simulink model "Triple_rotor_Tilerotor_model"  (R2024b)
settings: Solver=ode45  StartTime=0.0  StopTime=100  FixedStep=1e-3  RelTol=1e-3
values from neighbouring files (symbols this model uses):
  para =     [Triple_Rotors_Tilrotor_Parameters.mat]
undefined symbols (not defined in the file or in its folder): initial_height, initial_pitch, initial_vx, magnitude, rot2
libraries: simulink x9, slpidlib x5, matrix_library x4, vrlib x1
(part 1 of 3)
settings Model: Creator=18336  LastModifiedBy=18336
settings OptimizationCC: ReuseModelBlockBuffer=off
settings RTWCC: GPUComputeCapability=3.5

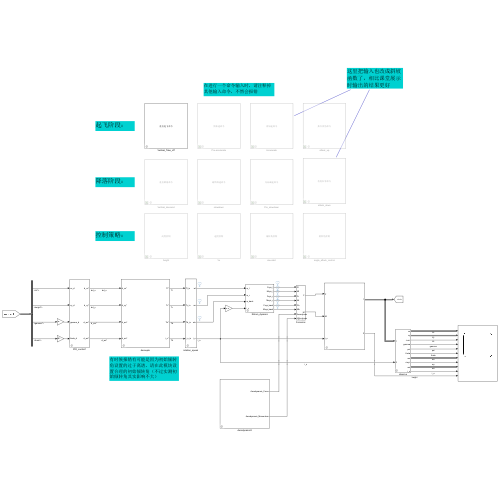
[thumbnail: Simulink's stored preview of the top-level diagram]
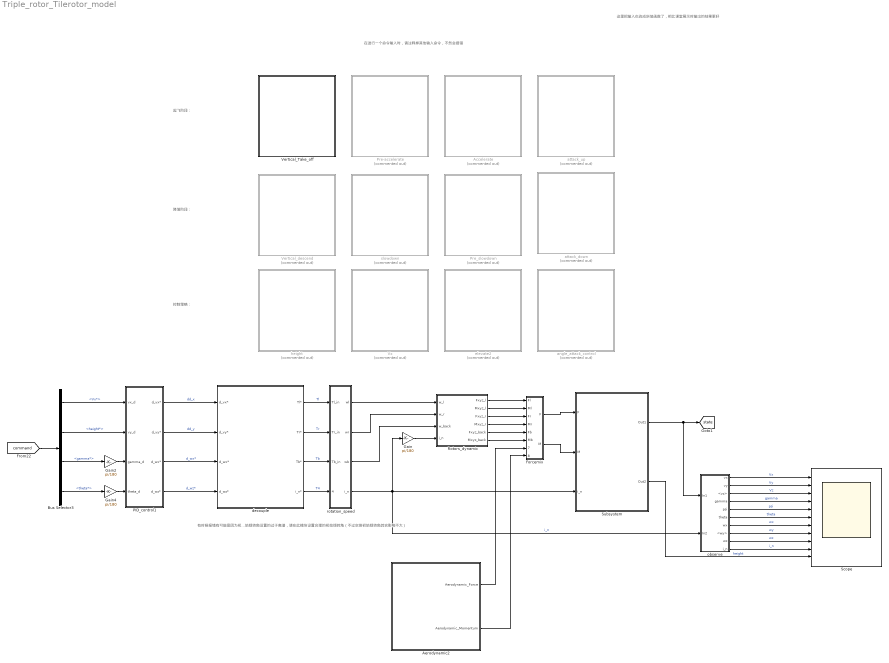
== system Triple_rotor_Tilerotor_model ==
  note: 这里把输入也改成斜坡函数了，相比课堂展示时输出的结果更好
  note: 在进行一个命令输入时，请注释掉其他输入命令，不然会报错
  note: 有时候报错有可能是因为初始倾转角设置的过于离谱，请在此模块设置合理的初始倾转角（不过实测初始倾转角其实影响不大）
  note: 起飞阶段：
  note: 降落阶段：
  note: 控制策略：
  Accelerate : Subsystem  Commented=on  mask{final_velocity=100, slope=10, Aerodynamic_switch=1}
      mask prompts: final_velocity "最终速度（m/s）"; slope "输入斜率"; Aerodynamic_switch "气动开关"
      mask DialogControl ParameterGroupVar Prompt: 参数
      mask Display: disp('再加速命令');
  Aerodynamic2 : Subsystem
  Bus Selector3 : BusSelector  OutputSignals=Vx*,height*,gamma*,theta*
  Forcemix : Subsystem
  Gain : Gain  Gain=pi/180
  Gain2 : Gain  Gain=pi/180
  Gain4 : Gain  Gain=pi/180
  PID_control1 : Subsystem  mask{P_d_vx=2, I_d_vx=1.3, D_d_vx=0, P_y=0.6, P_d_vy=1, I_d_vy=1.4, D_d_vy=0.1, P_wx=1, P_d_wx=1, I_d_wx=0, D_d_wx=0, P_wz=8, I_wz=2, D_wz=0, P_d_wz=6, I_d_wz=2, D_d_wz=8}
      mask prompts: P_d_vx "位置增益"; I_d_vx "积分增益"; D_d_vx "微分增益"; P_y "位置增益"; P_d_vy "速度位置增益"; I_d_vy "速度积分增益"; D_d_vy "速度微分增益"; P_wx "位置增益"; P_d_wx "二级位置增益"; I_d_wx "二级积分增益"; D_d_wx "二级微分增益"; P_wz "位置增益"; I_wz "积分增益"; D_wz "微分增益"; P_d_wz "二级位置增益"; I_d_wz "二级积分增益"; D_d_wz "二级微分增益"
      mask DialogControl ParameterGroupVar Prompt: 参数
      mask DialogControl x Prompt: x方向速度控制参数
      mask DialogControl y Prompt: y方向速度控制参数
      mask DialogControl wx Prompt: x方向角速度控制参数
      mask DialogControl wz Prompt: z方向角速度控制参数
  Pre-accelerate : Subsystem  Commented=on  mask{final_velocity=30, Aerodynamic_switch=0}
      mask prompts: final_velocity "最终速度（m/s）"; Aerodynamic_switch "气动开关"
      mask DialogControl ParameterGroupVar Prompt: 参数
      mask Display: disp('预加速命令');
  Pre_slowdown : Subsystem  Commented=on  mask{initial_velocity=100, Aerodynamic_switch=1}
      mask prompts: initial_velocity "初始速度（m/s）"; Aerodynamic_switch "气动开关"
      mask DialogControl ParameterGroupVar Prompt: 参数
      mask Display: disp('反向减速命令');
  Rotors_dynamic : Subsystem
  Scope : Scope  NumInputPorts=11
  Subsystem : Subsystem
  Vertical_Take_off : Subsystem  mask{slope_y=20, max_y=1000, Aerodynamic_switch=0}
      mask prompts: slope_y "上升速度（m/s）"; max_y "最终高度（m）"; Aerodynamic_switch "气动开关"
      mask DialogControl ParameterGroupVar Prompt: 参数
      mask Display: disp('垂直起飞命令');
  Vertical_descend : Subsystem  Commented=on  mask{slope_y=20, initial_y=1000, Aerodynamic_switch=0}
      mask prompts: slope_y "下降速度（m/s）"; initial_y "初始高度（m）"; Aerodynamic_switch "气动开关"
      mask DialogControl ParameterGroupVar Prompt: 参数
      mask Display: disp('垂直降落命令');
  Vx : Subsystem  Commented=on  mask{final_velocity=110, slope=10, Aerodynamic_switch=1}
      mask prompts: final_velocity "最终速度（m/s）"; slope "斜率"; Aerodynamic_switch "气动开关"
      mask DialogControl ParameterGroupVar Prompt: 参数
      mask Display: disp('速度控制');
  angle_attack_control : Subsystem  Commented=on  mask{final_theta=-2, slope=-2, Aerodynamic_switch=1}
      mask prompts: final_theta "最终俯仰角度"; slope "斜率"; Aerodynamic_switch "气动开关"
      mask DialogControl ParameterGroupVar Prompt: 参数
      mask Display: disp('俯仰角控制');
  attack_down : Subsystem  Commented=on  mask{initial_theta=4, slope=-1, Aerodynamic_switch=1}
      mask prompts: initial_theta "初始俯仰角"; slope "输入斜率"; Aerodynamic_switch "气动开关"
      mask DialogControl ParameterGroupVar Prompt: 参数
      mask Display: disp('攻角归零命令');
  attack_up : Subsystem  Commented=on  mask{final_theta=4, Aerodynamic_switch=1}
      mask prompts: final_theta "最终俯仰角"; Aerodynamic_switch "气动开关"
      mask DialogControl ParameterGroupVar Prompt: 参数
      mask Display: disp('抬升攻角命令');
  decouple : Subsystem  mask{initial_i_n=30}
      mask prompts: initial_i_n "初始短仓角"
      mask DialogControl ParameterGroupVar Prompt: 参数
  elevate2 : Subsystem  Commented=on  mask{max_gamma=4, slope=8, Aerodynamic_switch=0}
      mask prompts: max_gamma "最大滚转角°"; slope "斜率"; Aerodynamic_switch "气动开关"
      mask DialogControl ParameterGroupVar Prompt: 参数
      mask Display: disp('滚转角控制');
  height : Subsystem  Commented=on  mask{final_y=1100, slope=10, Aerodynamic_switch=1}
      mask prompts: final_y "最终高度"; slope "变化速度"; Aerodynamic_switch "气动开关"
      mask DialogControl ParameterGroupVar Prompt: 参数
      mask Display: disp('高度控制');
  observe : Subsystem
  rotation_speed : Subsystem  mask{maxrot=para.maxrot, minrot=1, maxi_n=170, mini_n=10}
      mask prompts: maxrot "旋翼最大转速"; minrot "旋翼最小转速"
      mask DialogControl ParameterGroupVar Prompt: 参数
  slowdown : Subsystem  Commented=on  mask{initial_velocity=30, Aerodynamic_switch=0}
      mask prompts: initial_velocity "初始速度（m/s）"; Aerodynamic_switch "气动开关"
      mask DialogControl ParameterGroupVar Prompt: 参数
      mask Display: disp('最终降速命令');
  tag scope: state=global
  wires:
  Subsystem/1(Out1) -> observe/1(In1), [state]
  rotation_speed/4(i_n) -> observe/2(In2), Subsystem/3(i_n), Gain/1  "i_n"
  Gain/1 -> Rotors_dynamic/4(i_n)
  Bus Selector3/2 -> PID_control1/2(vy_d)  "<height*>"
  PID_control1/1(d_vx*) -> decouple/1(d_vx*)  "dd_x"
  PID_control1/2(d_vy*) -> decouple/2(d_vy*)  "dd_y"
  PID_control1/3(d_wx*) -> decouple/3(d_wx*)  "d_wx*"
  PID_control1/4(d_wz*) -> decouple/4(d_wz*)  "d_wz*"
  Rotors_dynamic/4(Mxyz_r) -> Forcemix/4(Mr)
  Rotors_dynamic/1(Fxyz_l) -> Forcemix/1(Fl)
  Rotors_dynamic/2(Mxyz_l) -> Forcemix/2(Ml)
  Rotors_dynamic/6(Mxyz_back) -> Forcemix/6(Mb)
  rotation_speed/1(wl) -> Rotors_dynamic/1(w_l)
  rotation_speed/2(wr) -> Rotors_dynamic/2(w_r)
  rotation_speed/3(wb) -> Rotors_dynamic/3(w_back)
  Forcemix/1(F) -> Subsystem/1(F)
  Bus Selector3/3 -> Gain2/1  "<gamma*>"
  Rotors_dynamic/3(Fxyz_r) -> Forcemix/3(Fr)
  Rotors_dynamic/5(Fxyz_back) -> Forcemix/5(Fb)
  Aerodynamic2/1(Aerodynamic_Force) -> Forcemix/7(Aerodynamic_Force)
  Aerodynamic2/2(Aerodynamic_Momentum) -> Forcemix/8(Aerodynamic_Momentum)
  Gain4/1 -> PID_control1/4(theta_d)
  Forcemix/2(M) -> Subsystem/2(M)
  decouple/3(Tb*) -> rotation_speed/3(Tb_in)  "Tb"
  decouple/2(Tr*) -> rotation_speed/2(Tr_in)  "Tr"
  decouple/1(Tl*) -> rotation_speed/1(Tl_in)  "Tl"
  decouple/4(i_n*) -> rotation_speed/4(i_n_in)  "T4"
  Gain2/1 -> PID_control1/3(gamma_d)
  Subsystem/2(Out2) -> Scope/11  "height"
  [command] -> Bus Selector3/1
  Bus Selector3/1 -> PID_control1/1(vx_d)  "<Vx*>"
  Bus Selector3/4 -> Gain4/1  "<theta*>"
  observe/1(vx) -> Scope/1  "Vx"
  observe/2(vy) -> Scope/2  "Vy"
  observe/3(<vz>) -> Scope/3  "Vz"
  observe/4(gamma) -> Scope/4  "gamma"
  observe/5(psi) -> Scope/5  "psi"
  observe/6(theta) -> Scope/6  "theta"
  observe/7(wx) -> Scope/7  "wx"
  observe/8(<wy>) -> Scope/8  "wy"
  observe/9(wz) -> Scope/9  "wz"
  observe/10(i_n) -> Scope/10  "i_n"

== system Triple_rotor_Tilerotor_model/Accelerate ==
  note: 阶跃输入请用这个
  Bus Creator : BusCreator  Inputs=4
  Constant : Constant  Value=Aerodynamic_switch
  Constant1 : Constant  Value=0
  Constant2 : Constant  Value=1000
  Constant3 : Constant  Value=0
  Constant4 : Constant  Value=30
  Ramp : simulink/Sources/Ramp  slope=slope  start=0  InitialOutput=30
  Saturation2 : Saturate  UpperLimit=final_velocity  LowerLimit=0
  Step : Step  Commented=on  Time=0  Before=30  After=final_velocity  SampleTime=0
  gamma* : Constant  Value=0
  height : Constant  Value=1000
  theta* : Constant  Value=0
  tag scope: Aerodynamic_switch=global, command=global, initial_Vx=global, initial_gamma=global, initial_height=global, initial_theta=global
  wires:
  theta*/1 -> Bus Creator/4  "theta*"
  height/1 -> Bus Creator/2  "height*"
  gamma*/1 -> Bus Creator/3  "gamma*"
  Saturation2/1 -> Bus Creator/1  "Vx*"
  Bus Creator/1 -> [command]
  Constant/1 -> [Aerodynamic_switch]
  Constant1/1 -> [initial_theta]
  Constant3/1 -> [initial_gamma]
  Constant2/1 -> [initial_height]
  Constant4/1 -> [initial_Vx]
  Ramp/1 -> Saturation2/1

== system Triple_rotor_Tilerotor_model/Aerodynamic2 ==
  Aerodynamic Modal of Horizontal Stabilizer : Subsystem
  Aerodynamic Modal of the Left Verticall Stabilizer : Subsystem
  Aerodynamic Modal of the Right Verticall Stabilizer : Subsystem
  Aerodynamic Model of the Fuselage : Subsystem
  Aerodynamic Model of the Wing : Subsystem
  Demux{,1..3} (4 alike) : Demux  Outputs=3
  Product : Product
  Product1 : Product
  Resultant Force : Sum  Inputs=+++++
  Resultant Moment : Sum  Inputs=+++++
  Scope1 : Scope  NumInputPorts=3
  Scope2 : Scope  NumInputPorts=3
  Aerodynamic_Force : Outport
  Aerodynamic_Momentum : Outport  Port=2
  tag scope: Fx_forward=global, Fy_forward=global, Mx_forward=global, Mz_forward=global
  wires:
  [state] -> Aerodynamic Model of the Wing/1(In1)
  [state] -> Aerodynamic Model of the Fuselage/1(In1)
  Aerodynamic Modal of Horizontal Stabilizer/2(Vector of Momentum in Center of Gravity) -> Resultant Moment/3
  Aerodynamic Model of the Wing/2(Momentum of Wing Output) -> Resultant Moment/1
  Aerodynamic Modal of the Right Verticall Stabilizer/1(Out1) -> Resultant Force/5
  Aerodynamic Model of the Fuselage/1(Force of Fuselage) -> Resultant Force/3
  [state] -> Aerodynamic Modal of the Left Verticall Stabilizer/1(In1)
  Aerodynamic Modal of Horizontal Stabilizer/1(Vector of Force in Center of Gravity) -> Resultant Force/1
  [state] -> Aerodynamic Modal of the Right Verticall Stabilizer/1(In1)
  Aerodynamic Modal of the Right Verticall Stabilizer/2(Out2) -> Resultant Moment/5
  Aerodynamic Modal of the Left Verticall Stabilizer/2(Out2) -> Resultant Moment/4
  [state] -> Aerodynamic Modal of Horizontal Stabilizer/1(In1)
  Aerodynamic Modal of the Left Verticall Stabilizer/1(Out1) -> Resultant Force/4
  Aerodynamic Model of the Fuselage/2(Momentum of Fuselage) -> Resultant Moment/2
  Aerodynamic Model of the Wing/1(Force of Wing Output) -> Resultant Force/2
  Product/1 -> Demux2/1, Demux/1, Aerodynamic_Force/1
  Demux/1 -> [Fx_forward]
  Demux/2 -> [Fy_forward]
  Demux1/1 -> [Mx_forward]
  Demux1/3 -> [Mz_forward]
  Resultant Force/1 -> Product/1
  Resultant Moment/1 -> Product1/1
  Demux2/1 -> Scope1/1
  Demux2/2 -> Scope1/2
  Demux2/3 -> Scope1/3
  Demux3/1 -> Scope2/1
  Demux3/2 -> Scope2/2
  Product1/1 -> Demux3/1, Demux1/1, Aerodynamic_Momentum/1
  Demux3/3 -> Scope2/3
  [Aerodynamic_switch] -> Product1/2, Product/2

== system Triple_rotor_Tilerotor_model/Forcemix ==
  Fl : Inport
  Ml : Inport  Port=2
  Fr : Inport  Port=3
  Mr : Inport  Port=4
  Fb : Inport  Port=5
  Mb : Inport  Port=6
  Aerodynamic_Force : Inport  Port=7
  Aerodynamic_Momentum : Inport  Port=8
  Demux : Demux  Outputs=3
  Demux1 : Demux  Outputs=3
  Goto : Goto  Commented=on  GotoTag=F  TagVisibility=global
  Goto1 : Goto  Commented=on  GotoTag=M
  Scope1 : Scope  NumInputPorts=6
  rotor_forcemix : Subsystem
  F : Outport
  M : Outport  Port=2
  wires:
  Demux1/3 -> Scope1/6  "Mz"
  Demux1/1 -> Scope1/4  "Mx"
  Demux1/2 -> Scope1/5  "My"
  Demux/1 -> Scope1/1  "Fx"
  Demux/2 -> Scope1/2  "Fy"
  Demux/3 -> Scope1/3  "Fz"
  Fr/1 -> rotor_forcemix/3(Fr)
  Mr/1 -> rotor_forcemix/4(Mr)
  Fl/1 -> rotor_forcemix/1(Fl)
  Ml/1 -> rotor_forcemix/2(Ml)
  Fb/1 -> rotor_forcemix/5(Fb)
  Mb/1 -> rotor_forcemix/6(Mb)
  rotor_forcemix/1(Out1) -> F/1, Demux/1
  rotor_forcemix/2(Out2) -> Demux1/1, M/1
  Aerodynamic_Force/1 -> rotor_forcemix/7(AF)
  Aerodynamic_Momentum/1 -> rotor_forcemix/8(AM)

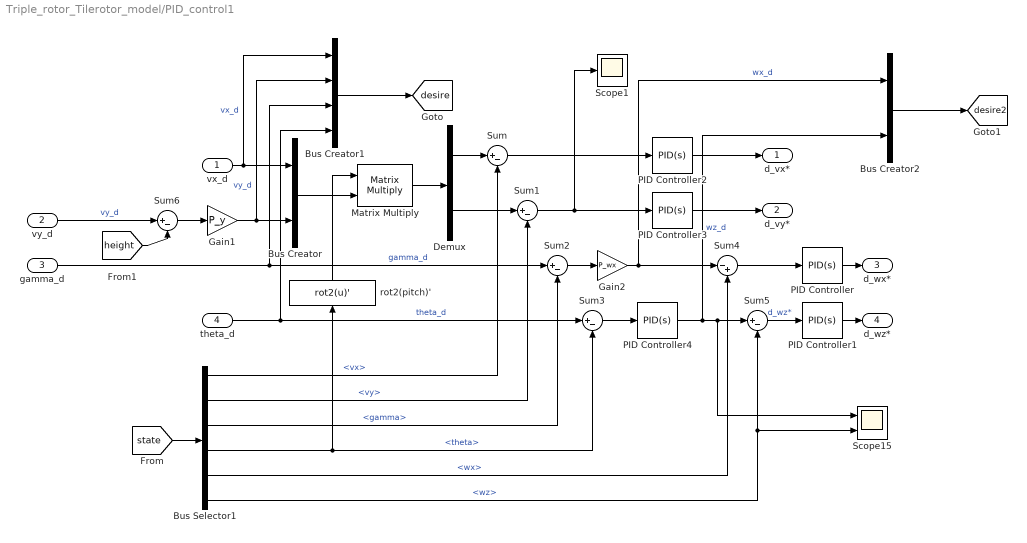
== system Triple_rotor_Tilerotor_model/PID_control1 ==
  vx_d : Inport
  vy_d : Inport  Port=2
  gamma_d : Inport  Port=3
  theta_d : Inport  Port=4
  Bus Creator : BusCreator  Inputs=2
  Bus Creator1 : BusCreator  Inputs=4
  Bus Creator2 : BusCreator  Inputs=2
  Bus Selector1 : BusSelector  OutputSignals=vx,vy,gamma,theta,wx,wz
  Demux : Demux  Outputs=2
  Gain1 : Gain  Gain=P_y
  Gain2 : Gain  Gain=P_wx
  Matrix Multiply : Product  Multiplication=Matrix(*)
  PID Controller : slpidlib/PID Controller  Controller=PID  Form=Parallel  TimeDomain=Continuous-time  UseExternalTs=off  SampleTime=-1  IntegratorMethod=Forward Euler  FilterMethod=Forward Euler  ControllerParametersSource=internal  P=P_d_wx  I=I_d_wx  UseKiTs=off  D=D_d_wx  UseExternalDerivativeSource=off  N=100  UseFilter=on  TunerSelectOption=Transfer Function Based (PID Tuner App)  InitialConditionSource=internal  InitialConditionForIntegrator=0  InitialConditionForFilter=0  DifferentiatorICPrevScaledInput=0  ExternalReset=none  TrackingMode=off  Kt=1  LimitOutput=off  SatLimitsSource=internal  UpperSaturationLimit=inf  LowerSaturationLimit=-inf  LinearizeAsGain=on  AntiWindupMode=none  Kb=1  LimitIntegrator=off  UpperIntegratorSaturationLimit=inf  LowerIntegratorSaturationLimit=-inf  POutMin=[]  POutMax=[]  IOutMin=[]  IOutMax=[]  DOutMin=[]  DOutMax=[]  NOutMin=[]  NOutMax=[]  SumOutMin=[]  SumOutMax=[]  SaturationOutMin=[]  SaturationOutMax=[]  PParamMin=[]  PParamMax=[]  IParamMin=[]  IParamMax=[]  DParamMin=[]  DParamMax=[]  NParamMin=[]  NParamMax=[]  KbParamMin=[]  KbParamMax=[]  KtParamMin=[]  KtParamMax=[]  KbOutMin=[]  KbOutMax=[]  KtOutMin=[]  KtOutMax=[]  IntegratorOutMin=[]  IntegratorOutMax=[]  FilterOutMin=[]  FilterOutMax=[]  SumI1OutMin=[]  SumI1OutMax=[]  SumI2OutMin=[]  SumI2OutMax=[]  SumI3OutMin=[]  SumI3OutMax=[]  SumI4OutMin=[]  SumI4OutMax=[]  SumDOutMin=[]  SumDOutMax=[]  DifferentiatorOutMin=[]  DifferentiatorOutMax=[]  FilterDiffOutCoefMin=[]  FilterDiffOutCoefMax=[]  ReciprocalOutMin=[]  ReciprocalOutMax=[]  SumDenOutMin=[]  SumDenOutMax=[]  SumNumOutMin=[]  SumNumOutMax=[]  DivideOutMin=[]  DivideOutMax=[]  UdiffTsProdOutMin=[]  UdiffTsProdOutMax=[]  NTsProdOutMin=[]  NTsProdOutMax=[]  UintegralTsProdOutMin=[]  UintegralTsProdOutMax=[]  UngainTsProdOutMin=[]  UngainTsProdOutMax=[]  ClampingZeroOutDataTypeStr=Inherit: Inherit via back propagation  ClampingZeroOutMin=[]  ClampingZeroOutMax=[]  FilterDenConstantOutDataTypeStr=Inherit: Inherit via back propagation  FilterDenConstantOutMin=[]  FilterDenConstantOutMax=[]  PCopyOutDataTypeStr=Inherit: Inherit via back propagation  PCopyOutMin=[]  PCopyOutMax=[]  NCopyOutDataTypeStr=Inherit: Inherit via back propagation  NCopyOutMin=[]  NCopyOutMax=[]  IntegratorContinuousStateAttributes=''  IntegratorStateMustResolveToSignalObject=off  IntegratorRTWStateStorageClass=Auto  FilterContinuousStateAttributes=''  FilterStateMustResolveToSignalObject=off  FilterRTWStateStorageClass=Auto  ParallelPVariant=InternalParameters  IdealPVariant=Disabled  IVariant=InternalParameters  DVariant=InternalParameters  IntegratorVariant=Continuous  SatVariant=Disabled  AWVariant=Passthrough  PCopyVariant=Disabled  TRVariant=Disabled  FdbkBlocksVariant=Forward  IdealPFdbkVariant=Disabled  SatFdbkVariant=Disabled  DerivativeFilterVariant=ContFilter  NVariant=InternalParameters  NCopyVariant=Disabled  FilterICVariant=InternalICsFilter  IntegratorICVariant=InternalICs  ExternalResetVariant=Disabled  TRSumVariant=Passthrough  SumFdbkVariant=Disabled  SumVariant=Sum_PID  TsampFilterVariant=InternalTs  TsampNgainVariant=Passthrough  TsampIntegralVariant=Disabled_SignalSpec  ExternalSaturationOutDataTypeStr=Inherit: Same as second input  DerivativeSourceVariant=ErrorSignal  PreIntVariant=InternalPreInt
  PID Controller1 : slpidlib/PID Controller  Controller=PID  Form=Parallel  TimeDomain=Continuous-time  UseExternalTs=off  SampleTime=-1  IntegratorMethod=Forward Euler  FilterMethod=Forward Euler  ControllerParametersSource=internal  P=P_d_wz  I=I_d_wz  UseKiTs=off  D=D_d_wz  UseExternalDerivativeSource=off  N=100  UseFilter=on  TunerSelectOption=Transfer Function Based (PID Tuner App)  InitialConditionSource=internal  InitialConditionForIntegrator=0  InitialConditionForFilter=0  DifferentiatorICPrevScaledInput=0  ExternalReset=none  TrackingMode=off  Kt=1  LimitOutput=off  SatLimitsSource=internal  UpperSaturationLimit=inf  LowerSaturationLimit=-inf  LinearizeAsGain=on  AntiWindupMode=none  Kb=1  LimitIntegrator=off  UpperIntegratorSaturationLimit=inf  LowerIntegratorSaturationLimit=-inf  POutMin=[]  POutMax=[]  IOutMin=[]  IOutMax=[]  DOutMin=[]  DOutMax=[]  NOutMin=[]  NOutMax=[]  SumOutMin=[]  SumOutMax=[]  SaturationOutMin=[]  SaturationOutMax=[]  PParamMin=[]  PParamMax=[]  IParamMin=[]  IParamMax=[]  DParamMin=[]  DParamMax=[]  NParamMin=[]  NParamMax=[]  KbParamMin=[]  KbParamMax=[]  KtParamMin=[]  KtParamMax=[]  KbOutMin=[]  KbOutMax=[]  KtOutMin=[]  KtOutMax=[]  IntegratorOutMin=[]  IntegratorOutMax=[]  FilterOutMin=[]  FilterOutMax=[]  SumI1OutMin=[]  SumI1OutMax=[]  SumI2OutMin=[]  SumI2OutMax=[]  SumI3OutMin=[]  SumI3OutMax=[]  SumI4OutMin=[]  SumI4OutMax=[]  SumDOutMin=[]  SumDOutMax=[]  DifferentiatorOutMin=[]  DifferentiatorOutMax=[]  FilterDiffOutCoefMin=[]  FilterDiffOutCoefMax=[]  ReciprocalOutMin=[]  ReciprocalOutMax=[]  SumDenOutMin=[]  SumDenOutMax=[]  SumNumOutMin=[]  SumNumOutMax=[]  DivideOutMin=[]  DivideOutMax=[]  UdiffTsProdOutMin=[]  UdiffTsProdOutMax=[]  NTsProdOutMin=[]  NTsProdOutMax=[]  UintegralTsProdOutMin=[]  UintegralTsProdOutMax=[]  UngainTsProdOutMin=[]  UngainTsProdOutMax=[]  ClampingZeroOutDataTypeStr=Inherit: Inherit via back propagation  ClampingZeroOutMin=[]  ClampingZeroOutMax=[]  FilterDenConstantOutDataTypeStr=Inherit: Inherit via back propagation  FilterDenConstantOutMin=[]  FilterDenConstantOutMax=[]  PCopyOutDataTypeStr=Inherit: Inherit via back propagation  PCopyOutMin=[]  PCopyOutMax=[]  NCopyOutDataTypeStr=Inherit: Inherit via back propagation  NCopyOutMin=[]  NCopyOutMax=[]  IntegratorContinuousStateAttributes=''  IntegratorStateMustResolveToSignalObject=off  IntegratorRTWStateStorageClass=Auto  FilterContinuousStateAttributes=''  FilterStateMustResolveToSignalObject=off  FilterRTWStateStorageClass=Auto  ParallelPVariant=InternalParameters  IdealPVariant=Disabled  IVariant=InternalParameters  DVariant=InternalParameters  IntegratorVariant=Continuous  SatVariant=Disabled  AWVariant=Passthrough  PCopyVariant=Disabled  TRVariant=Disabled  FdbkBlocksVariant=Forward  IdealPFdbkVariant=Disabled  SatFdbkVariant=Disabled  DerivativeFilterVariant=ContFilter  NVariant=InternalParameters  NCopyVariant=Disabled  FilterICVariant=InternalICsFilter  IntegratorICVariant=InternalICs  ExternalResetVariant=Disabled  TRSumVariant=Passthrough  SumFdbkVariant=Disabled  SumVariant=Sum_PID  TsampFilterVariant=InternalTs  TsampNgainVariant=Passthrough  TsampIntegralVariant=Disabled_SignalSpec  ExternalSaturationOutDataTypeStr=Inherit: Same as second input  DerivativeSourceVariant=ErrorSignal  PreIntVariant=InternalPreInt
  PID Controller2 : slpidlib/PID Controller  Controller=PID  Form=Parallel  TimeDomain=Continuous-time  UseExternalTs=off  SampleTime=-1  IntegratorMethod=Forward Euler  FilterMethod=Forward Euler  ControllerParametersSource=internal  P=P_d_vx  I=I_d_vx  UseKiTs=off  D=D_d_vx  UseExternalDerivativeSource=off  N=100  UseFilter=on  TunerSelectOption=Transfer Function Based (PID Tuner App)  InitialConditionSource=internal  InitialConditionForIntegrator=0  InitialConditionForFilter=0  DifferentiatorICPrevScaledInput=0  ExternalReset=none  TrackingMode=off  Kt=1  LimitOutput=off  SatLimitsSource=internal  UpperSaturationLimit=inf  LowerSaturationLimit=-inf  LinearizeAsGain=on  AntiWindupMode=none  Kb=1  LimitIntegrator=off  UpperIntegratorSaturationLimit=inf  LowerIntegratorSaturationLimit=-inf  POutMin=[]  POutMax=[]  IOutMin=[]  IOutMax=[]  DOutMin=[]  DOutMax=[]  NOutMin=[]  NOutMax=[]  SumOutMin=[]  SumOutMax=[]  SaturationOutMin=[]  SaturationOutMax=[]  PParamMin=[]  PParamMax=[]  IParamMin=[]  IParamMax=[]  DParamMin=[]  DParamMax=[]  NParamMin=[]  NParamMax=[]  KbParamMin=[]  KbParamMax=[]  KtParamMin=[]  KtParamMax=[]  KbOutMin=[]  KbOutMax=[]  KtOutMin=[]  KtOutMax=[]  IntegratorOutMin=[]  IntegratorOutMax=[]  FilterOutMin=[]  FilterOutMax=[]  SumI1OutMin=[]  SumI1OutMax=[]  SumI2OutMin=[]  SumI2OutMax=[]  SumI3OutMin=[]  SumI3OutMax=[]  SumI4OutMin=[]  SumI4OutMax=[]  SumDOutMin=[]  SumDOutMax=[]  DifferentiatorOutMin=[]  DifferentiatorOutMax=[]  FilterDiffOutCoefMin=[]  FilterDiffOutCoefMax=[]  ReciprocalOutMin=[]  ReciprocalOutMax=[]  SumDenOutMin=[]  SumDenOutMax=[]  SumNumOutMin=[]  SumNumOutMax=[]  DivideOutMin=[]  DivideOutMax=[]  UdiffTsProdOutMin=[]  UdiffTsProdOutMax=[]  NTsProdOutMin=[]  NTsProdOutMax=[]  UintegralTsProdOutMin=[]  UintegralTsProdOutMax=[]  UngainTsProdOutMin=[]  UngainTsProdOutMax=[]  ClampingZeroOutDataTypeStr=Inherit: Inherit via back propagation  ClampingZeroOutMin=[]  ClampingZeroOutMax=[]  FilterDenConstantOutDataTypeStr=Inherit: Inherit via back propagation  FilterDenConstantOutMin=[]  FilterDenConstantOutMax=[]  PCopyOutDataTypeStr=Inherit: Inherit via back propagation  PCopyOutMin=[]  PCopyOutMax=[]  NCopyOutDataTypeStr=Inherit: Inherit via back propagation  NCopyOutMin=[]  NCopyOutMax=[]  IntegratorContinuousStateAttributes=''  IntegratorStateMustResolveToSignalObject=off  IntegratorRTWStateStorageClass=Auto  FilterContinuousStateAttributes=''  FilterStateMustResolveToSignalObject=off  FilterRTWStateStorageClass=Auto  ParallelPVariant=InternalParameters  IdealPVariant=Disabled  IVariant=InternalParameters  DVariant=InternalParameters  IntegratorVariant=Continuous  SatVariant=Disabled  AWVariant=Passthrough  PCopyVariant=Disabled  TRVariant=Disabled  FdbkBlocksVariant=Forward  IdealPFdbkVariant=Disabled  SatFdbkVariant=Disabled  DerivativeFilterVariant=ContFilter  NVariant=InternalParameters  NCopyVariant=Disabled  FilterICVariant=InternalICsFilter  IntegratorICVariant=InternalICs  ExternalResetVariant=Disabled  TRSumVariant=Passthrough  SumFdbkVariant=Disabled  SumVariant=Sum_PID  TsampFilterVariant=InternalTs  TsampNgainVariant=Passthrough  TsampIntegralVariant=Disabled_SignalSpec  ExternalSaturationOutDataTypeStr=Inherit: Same as second input  DerivativeSourceVariant=ErrorSignal  PreIntVariant=InternalPreInt
  PID Controller3 : slpidlib/PID Controller  Controller=PID  Form=Parallel  TimeDomain=Continuous-time  UseExternalTs=off  SampleTime=-1  IntegratorMethod=Forward Euler  FilterMethod=Forward Euler  ControllerParametersSource=internal  P=P_d_vy  I=I_d_vy  UseKiTs=off  D=D_d_vy  UseExternalDerivativeSource=off  N=100  UseFilter=on  TunerSelectOption=Transfer Function Based (PID Tuner App)  InitialConditionSource=internal  InitialConditionForIntegrator=0  InitialConditionForFilter=0  DifferentiatorICPrevScaledInput=0  ExternalReset=none  TrackingMode=off  Kt=1  LimitOutput=off  SatLimitsSource=internal  UpperSaturationLimit=inf  LowerSaturationLimit=-inf  LinearizeAsGain=on  AntiWindupMode=none  Kb=1  LimitIntegrator=off  UpperIntegratorSaturationLimit=inf  LowerIntegratorSaturationLimit=-inf  POutMin=[]  POutMax=[]  IOutMin=[]  IOutMax=[]  DOutMin=[]  DOutMax=[]  NOutMin=[]  NOutMax=[]  SumOutMin=[]  SumOutMax=[]  SaturationOutMin=[]  SaturationOutMax=[]  PParamMin=[]  PParamMax=[]  IParamMin=[]  IParamMax=[]  DParamMin=[]  DParamMax=[]  NParamMin=[]  NParamMax=[]  KbParamMin=[]  KbParamMax=[]  KtParamMin=[]  KtParamMax=[]  KbOutMin=[]  KbOutMax=[]  KtOutMin=[]  KtOutMax=[]  IntegratorOutMin=[]  IntegratorOutMax=[]  FilterOutMin=[]  FilterOutMax=[]  SumI1OutMin=[]  SumI1OutMax=[]  SumI2OutMin=[]  SumI2OutMax=[]  SumI3OutMin=[]  SumI3OutMax=[]  SumI4OutMin=[]  SumI4OutMax=[]  SumDOutMin=[]  SumDOutMax=[]  DifferentiatorOutMin=[]  DifferentiatorOutMax=[]  FilterDiffOutCoefMin=[]  FilterDiffOutCoefMax=[]  ReciprocalOutMin=[]  ReciprocalOutMax=[]  SumDenOutMin=[]  SumDenOutMax=[]  SumNumOutMin=[]  SumNumOutMax=[]  DivideOutMin=[]  DivideOutMax=[]  UdiffTsProdOutMin=[]  UdiffTsProdOutMax=[]  NTsProdOutMin=[]  NTsProdOutMax=[]  UintegralTsProdOutMin=[]  UintegralTsProdOutMax=[]  UngainTsProdOutMin=[]  UngainTsProdOutMax=[]  ClampingZeroOutDataTypeStr=Inherit: Inherit via back propagation  ClampingZeroOutMin=[]  ClampingZeroOutMax=[]  FilterDenConstantOutDataTypeStr=Inherit: Inherit via back propagation  FilterDenConstantOutMin=[]  FilterDenConstantOutMax=[]  PCopyOutDataTypeStr=Inherit: Inherit via back propagation  PCopyOutMin=[]  PCopyOutMax=[]  NCopyOutDataTypeStr=Inherit: Inherit via back propagation  NCopyOutMin=[]  NCopyOutMax=[]  IntegratorContinuousStateAttributes=''  IntegratorStateMustResolveToSignalObject=off  IntegratorRTWStateStorageClass=Auto  FilterContinuousStateAttributes=''  FilterStateMustResolveToSignalObject=off  FilterRTWStateStorageClass=Auto  ParallelPVariant=InternalParameters  IdealPVariant=Disabled  IVariant=InternalParameters  DVariant=InternalParameters  IntegratorVariant=Continuous  SatVariant=Disabled  AWVariant=Passthrough  PCopyVariant=Disabled  TRVariant=Disabled  FdbkBlocksVariant=Forward  IdealPFdbkVariant=Disabled  SatFdbkVariant=Disabled  DerivativeFilterVariant=ContFilter  NVariant=InternalParameters  NCopyVariant=Disabled  FilterICVariant=InternalICsFilter  IntegratorICVariant=InternalICs  ExternalResetVariant=Disabled  TRSumVariant=Passthrough  SumFdbkVariant=Disabled  SumVariant=Sum_PID  TsampFilterVariant=InternalTs  TsampNgainVariant=Passthrough  TsampIntegralVariant=Disabled_SignalSpec  ExternalSaturationOutDataTypeStr=Inherit: Same as second input  DerivativeSourceVariant=ErrorSignal  PreIntVariant=InternalPreInt
  PID Controller4 : slpidlib/PID Controller  Controller=PID  Form=Parallel  TimeDomain=Continuous-time  UseExternalTs=off  SampleTime=-1  IntegratorMethod=Forward Euler  FilterMethod=Forward Euler  ControllerParametersSource=internal  P=P_wz  I=I_wz  UseKiTs=off  D=D_wz  UseExternalDerivativeSource=off  N=100  UseFilter=on  TunerSelectOption=Transfer Function Based (PID Tuner App)  InitialConditionSource=internal  InitialConditionForIntegrator=0  InitialConditionForFilter=0  DifferentiatorICPrevScaledInput=0  ExternalReset=none  TrackingMode=off  Kt=1  LimitOutput=off  SatLimitsSource=internal  UpperSaturationLimit=inf  LowerSaturationLimit=-inf  LinearizeAsGain=on  AntiWindupMode=none  Kb=1  LimitIntegrator=off  UpperIntegratorSaturationLimit=inf  LowerIntegratorSaturationLimit=-inf  POutMin=[]  POutMax=[]  IOutMin=[]  IOutMax=[]  DOutMin=[]  DOutMax=[]  NOutMin=[]  NOutMax=[]  SumOutMin=[]  SumOutMax=[]  SaturationOutMin=[]  SaturationOutMax=[]  PParamMin=[]  PParamMax=[]  IParamMin=[]  IParamMax=[]  DParamMin=[]  DParamMax=[]  NParamMin=[]  NParamMax=[]  KbParamMin=[]  KbParamMax=[]  KtParamMin=[]  KtParamMax=[]  KbOutMin=[]  KbOutMax=[]  KtOutMin=[]  KtOutMax=[]  IntegratorOutMin=[]  IntegratorOutMax=[]  FilterOutMin=[]  FilterOutMax=[]  SumI1OutMin=[]  SumI1OutMax=[]  SumI2OutMin=[]  SumI2OutMax=[]  SumI3OutMin=[]  SumI3OutMax=[]  SumI4OutMin=[]  SumI4OutMax=[]  SumDOutMin=[]  SumDOutMax=[]  DifferentiatorOutMin=[]  DifferentiatorOutMax=[]  FilterDiffOutCoefMin=[]  FilterDiffOutCoefMax=[]  ReciprocalOutMin=[]  ReciprocalOutMax=[]  SumDenOutMin=[]  SumDenOutMax=[]  SumNumOutMin=[]  SumNumOutMax=[]  DivideOutMin=[]  DivideOutMax=[]  UdiffTsProdOutMin=[]  UdiffTsProdOutMax=[]  NTsProdOutMin=[]  NTsProdOutMax=[]  UintegralTsProdOutMin=[]  UintegralTsProdOutMax=[]  UngainTsProdOutMin=[]  UngainTsProdOutMax=[]  ClampingZeroOutDataTypeStr=Inherit: Inherit via back propagation  ClampingZeroOutMin=[]  ClampingZeroOutMax=[]  FilterDenConstantOutDataTypeStr=Inherit: Inherit via back propagation  FilterDenConstantOutMin=[]  FilterDenConstantOutMax=[]  PCopyOutDataTypeStr=Inherit: Inherit via back propagation  PCopyOutMin=[]  PCopyOutMax=[]  NCopyOutDataTypeStr=Inherit: Inherit via back propagation  NCopyOutMin=[]  NCopyOutMax=[]  IntegratorContinuousStateAttributes=''  IntegratorStateMustResolveToSignalObject=off  IntegratorRTWStateStorageClass=Auto  FilterContinuousStateAttributes=''  FilterStateMustResolveToSignalObject=off  FilterRTWStateStorageClass=Auto  ParallelPVariant=InternalParameters  IdealPVariant=Disabled  IVariant=InternalParameters  DVariant=InternalParameters  IntegratorVariant=Continuous  SatVariant=Disabled  AWVariant=Passthrough  PCopyVariant=Disabled  TRVariant=Disabled  FdbkBlocksVariant=Forward  IdealPFdbkVariant=Disabled  SatFdbkVariant=Disabled  DerivativeFilterVariant=ContFilter  NVariant=InternalParameters  NCopyVariant=Disabled  FilterICVariant=InternalICsFilter  IntegratorICVariant=InternalICs  ExternalResetVariant=Disabled  TRSumVariant=Passthrough  SumFdbkVariant=Disabled  SumVariant=Sum_PID  TsampFilterVariant=InternalTs  TsampNgainVariant=Passthrough  TsampIntegralVariant=Disabled_SignalSpec  ExternalSaturationOutDataTypeStr=Inherit: Same as second input  DerivativeSourceVariant=ErrorSignal  PreIntVariant=InternalPreInt
  Scope1 : Scope
  Scope15 : Scope  NumInputPorts=2
  Sum{,1..3,5..6} (6 alike) : Sum  Inputs=|+-
  Sum4 : Sum  Inputs=|-+
  rot2(pitch)' : MATLABFcn  MATLABFcn=rot2(u)'  OutputDimensions=[2 2]  Output1D=off
  d_vx* : Outport
  d_vy* : Outport  Port=2
  d_wx* : Outport  Port=3
  d_wz* : Outport  Port=4
  tag scope: desire2=global, desire=global
  wires:
  Bus Selector1/3 -> Sum2/2  "<gamma>"
  PID Controller3/1 -> d_vy*/1
  Bus Selector1/5 -> Sum4/2  "<wx>"
  Sum3/1 -> PID Controller4/1
  Bus Selector1/1 -> Sum/2  "<vx>"
  Gain2/1 -> Sum4/1, Bus Creator2/1  "wx_d"
  Sum4/1 -> PID Controller/1
  rot2(pitch)'/1 -> Matrix Multiply/1
  PID Controller1/1 -> d_wz*/1
  PID Controller2/1 -> d_vx*/1
  Bus Selector1/2 -> Sum1/2  "<vy>"
  [state] -> Bus Selector1/1
  theta_d/1 -> Sum3/1, Bus Creator1/4  "theta_d"
  Sum/1 -> PID Controller2/1
  PID Controller/1 -> d_wx*/1
  vx_d/1 -> Bus Creator1/1, Bus Creator/1  "vx_d"
  Sum6/1 -> Gain1/1
  Bus Selector1/4 -> Sum3/2, rot2(pitch)'/1  "<theta>"
  Bus Creator/1 -> Matrix Multiply/2
  Matrix Multiply/1 -> Demux/1
  Demux/1 -> Sum/1
  Demux/2 -> Sum1/1
  Bus Selector1/6 -> Scope15/2, Sum5/2  "<wz>"
  Bus Creator1/1 -> [desire]
  Sum2/1 -> Gain2/1
  Bus Creator2/1 -> [desire2]
  PID Controller4/1 -> Scope15/1, Sum5/1, Bus Creator2/2  "wz_d"
  Sum5/1 -> PID Controller1/1  "d_wz*"
  Sum1/1 -> Scope1/1, PID Controller3/1
  gamma_d/1 -> Sum2/1, Bus Creator1/3  "gamma_d"
  [height] -> Sum6/2
  vy_d/1 -> Sum6/1  "vy_d"
  Gain1/1 -> Bus Creator1/2, Bus Creator/2  "vy_d"

== system Triple_rotor_Tilerotor_model/Pre-accelerate ==
  Bus Creator : BusCreator  Inputs=4
  Constant : Constant  Value=Aerodynamic_switch
  Constant1 : Constant  Value=0
  Constant2 : Constant  Value=1000
  Constant3 : Constant  Value=0
  Constant4 : Constant  Value=1e-5
  Step : Step  Time=0  After=final_velocity  SampleTime=0
  gamma* : Constant  Value=0
  height : Constant  Value=1000
  theta* : Constant  Value=0
  tag scope: Aerodynamic_switch=global, command=global, initial_Vx=global, initial_gamma=global, initial_height=global, initial_theta=global
  wires:
  theta*/1 -> Bus Creator/4  "theta*"
  height/1 -> Bus Creator/2  "height*"
  gamma*/1 -> Bus Creator/3  "gamma*"
  Step/1 -> Bus Creator/1  "Vx*"
  Bus Creator/1 -> [command]
  Constant/1 -> [Aerodynamic_switch]
  Constant1/1 -> [initial_theta]
  Constant3/1 -> [initial_gamma]
  Constant2/1 -> [initial_height]
  Constant4/1 -> [initial_Vx]

== system Triple_rotor_Tilerotor_model/Pre_slowdown ==
  Bus Creator : BusCreator  Inputs=4
  Constant : Constant  Value=Aerodynamic_switch
  Constant1 : Constant  Value=0
  Constant2 : Constant  Value=1000
  Constant3 : Constant  Value=0
  Constant4 : Constant  Value=initial_velocity
  Ramp : simulink/Sources/Ramp  slope=-(initial_velocity-30)/10  start=0  InitialOutput=initial_velocity
  Saturation2 : Saturate  UpperLimit=inf  LowerLimit=30
  gamma* : Constant  Value=0
  height : Constant  Value=1000
  theta* : Constant  Value=0
  tag scope: Aerodynamic_switch=global, command=global, initial_Vx=global, initial_gamma=global, initial_height=global, initial_theta=global
  wires:
  theta*/1 -> Bus Creator/4  "theta*"
  height/1 -> Bus Creator/2  "height*"
  gamma*/1 -> Bus Creator/3  "gamma*"
  Saturation2/1 -> Bus Creator/1  "Vx*"
  Bus Creator/1 -> [command]
  Constant/1 -> [Aerodynamic_switch]
  Constant1/1 -> [initial_theta]
  Constant3/1 -> [initial_gamma]
  Constant2/1 -> [initial_height]
  Constant4/1 -> [initial_Vx]
  Ramp/1 -> Saturation2/1

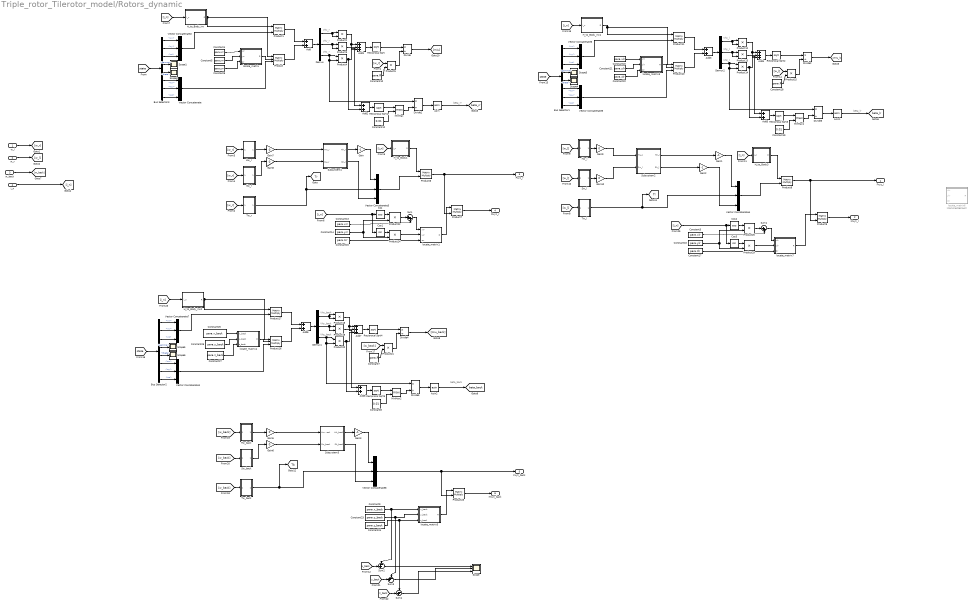
== system Triple_rotor_Tilerotor_model/Rotors_dynamic ==
  note: Vhx_r
  note: Vhx_l
  note: beta_lr
  note: beta_rr
  note: Vhz_l
  note: Vhz_back
  note: Vhy_r
  note: Vhy_l
  note: Vhz_r
  note: beta_back
  note: Vhx_back
  note: Vhy_back
  w_l : Inport
  w_r : Inport  Port=2
  w_back : Inport  Port=3
  i_n : Inport  Port=4
  Add{,2..3,5..6,8} (6 alike) : Sum
  Add1 : Sum  Inputs=+++
  Add4 : Sum  Inputs=+++
  Add7 : Sum  Inputs=+++
  Asin : Trigonometry  Operator=asin
  Asin1 : Trigonometry  Operator=asin
  Asin2 : Trigonometry  Operator=asin
  Bus Selector1 : BusSelector  OutputSignals=vx,vy,vz,gamma,theta,wx,wy,wz
  Bus Selector2 : BusSelector  OutputSignals=vx,vy,vz,gamma,theta,wx,wy,wz
  Bus Selector3 : BusSelector  OutputSignals=vx,vy,vz,gamma,theta,wx,wy,wz
  Constant10 : Constant  Value=para.R
  Constant12 : Constant  Value=0.01
  Constant13 : Constant  Value=para.xrr
  Constant14 : Constant  Value=para.yrr
  Constant15 : Constant  Value=para.zrr
  Constant16 : Constant  Value=para.ylr
  Constant17 : Constant  Value=para.zlr
  Constant18 : Constant  Value=para.R
  Constant19 : Constant  Value=0.01
  Constant20 : Constant  Value=para.xlr
  Constant21 : Constant  Value=para.ylr
  Constant22 : Constant  Value=para.zlr
  Constant23 : Constant  Value=para.y_back
  Constant24 : Constant  Value=para.z_back
  Constant25 : Constant  Value=para.x_back
  Constant26 : Constant  Value=para.y_back
  Constant27 : Constant  Value=para.z_back
  Constant3 : Constant  Value=para.xlr
  Constant4 : Constant  Value=para.xrr
  Constant5 : Constant  Value=para.yrr
  Constant6 : Constant  Value=para.zrr
  Constant7 : Constant  Value=para.R
  Constant8 : Constant  Value=0.01
  Constant9 : Constant  Value=para.x_back
  Cos : Trigonometry  Operator=cos
  Cos1 : Trigonometry
  Cos2 : Trigonometry  Operator=cos
  Cos3 : Trigonometry
  Demux : Demux  Outputs=3
  Demux1 : Demux  Outputs=3
  Demux2 : Demux  Outputs=3
  Divide{,1..5} (6 alike) : Product  Inputs=*/
  Gain{,1..3} (4 alike) : Gain  Gain=-1
  Gain{5..10} (6 alike) : Gain  Gain=0
  H_to_Body1 : MATLAB Function  TreatAsAtomicUnit=on
  H_to_Body3 : MATLAB Function  TreatAsAtomicUnit=on
  H_to_Body_inv : MATLAB Function  TreatAsAtomicUnit=on
  H_to_Body_inv1 : MATLAB Function  TreatAsAtomicUnit=on
  H_to_Body_inv2 : MATLAB Function  TreatAsAtomicUnit=on
  Hw_back : Subsystem
  Hw_l : Subsystem
  Hw_r : Subsystem
  MinMax : MinMax  Function=max  Inputs=2
  MinMax1 : MinMax  Function=max  Inputs=2
  MinMax2 : MinMax  Function=max  Inputs=2
  Product : Product  Inputs=3  Multiplication=Matrix(*)
  Product{1,6..9,11,17,23} (8 alike) : Product  Multiplication=Matrix(*)
  Product10 : Product  Inputs=3  Multiplication=Matrix(*)
  Product{2..5,12..15,18..22,24..25,29} (16 alike) : Product
  Product16 : Product  Inputs=3  Multiplication=Matrix(*)
  Reciprocal Sqrt{,1..5} (6 alike) : Sqrt
  Scope : Scope  NumInputPorts=3
  Scope{1..6} (6 alike) : Scope
  Subsystem1 : Subsystem
  Subsystem2 : Subsystem
  Subsystem3 : Subsystem
  Sum : Sum  Inputs=|++
  Sum1 : Sum  Inputs=|++
  Sum2 : Sum  Inputs=-+|
  Sum3 : Sum  Inputs=-+|
  Sum4 : Sum  Inputs=-+|
  Sw_back : Subsystem
  Sw_l : Subsystem
  Sw_r : Subsystem
  Tw_back : Subsystem
  Tw_l : Subsystem
  Tw_r : Subsystem
  Vector Concatenate{,1..8} (9 alike) : Concatenate  NumInputs=3  Mode=Multidimensional array
  locate_matrix : MATLAB Function  TreatAsAtomicUnit=on
  locate_matrix1 : MATLAB Function  TreatAsAtomicUnit=on
  locate_matrix3 : MATLAB Function  TreatAsAtomicUnit=on
  locate_matrix4 : MATLAB Function  TreatAsAtomicUnit=on
  locate_matrix5 : MATLAB Function  TreatAsAtomicUnit=on
  locate_matrix6 : MATLAB Function  Commented=on  TreatAsAtomicUnit=on
  locate_matrix7 : MATLAB Function  TreatAsAtomicUnit=on
  Fxyz_l : Outport
  Mxyz_l : Outport  Port=2
  Fxyz_r : Outport  Port=3
  Mxyz_r : Outport  Port=4
  Fxyz_back : Outport  Port=5
  Mxyz_back : Outport  Port=6
  tag scope: Tb=global, Tl=global, Tr=global, beta_back=global, beta_lr=global, beta_rr=global
  wires:
  Product3/1 -> Add1/2
  Bus Selector2/3 -> Vector Concatenate7/3  "<vz>"
  Constant5/1 -> locate_matrix/2(yrr)
  Demux1/1 -> Product18/2, Product18/1
  Constant7/1 -> Product21/2
  Demux2/1 -> Product12/2, Product12/1
  Constant26/1 -> locate_matrix4/2(y_back)
  Bus Selector1/3 -> Vector Concatenate6/3  "<vz>"
  [w_r] -> Sw_r/1(In1)
  [state] -> Bus Selector3/1
  Divide3/1 -> Asin1/1
  Product21/1 -> Divide4/2
  Add2/1 -> Reciprocal Sqrt1/1
  Product18/1 -> Add8/1, Add7/1
  Product16/1 -> Add6/2
  Constant10/1 -> Product5/2
  Product14/1 -> Add5/2, Add4/3
  Demux/3 -> Product4/1, Divide1/1, Product4/2
  H_to_Body_inv/1(R) -> Product1/1, Product/1
  [state] -> Bus Selector1/1
  Divide2/1 -> [miu_l]
  Product12/1 -> Add5/1, Add4/1
  Tw_l/1(Tw_l) -> [Tl], Vector Concatenate4/2
  Product8/1 -> Product9/2, Fxyz_l/1
  Product/1 -> Add/2
  Product2/1 -> Add2/1, Add1/1
  [w_r] -> Hw_r/1(In1)
  Subsystem3/1(Hh_back) -> Gain3/1
  Bus Selector2/8 -> Vector Concatenate1/3  "<wz>"
  Divide5/1 -> Asin2/1
  Add8/1 -> Reciprocal Sqrt5/1
  [w_back] -> Hw_back/1(In1)
  Add4/1 -> Reciprocal Sqrt2/1
  Demux/2 -> Product3/2, Product3/1
  locate_matrix3/1(R) -> Product10/2
  H_to_Body3/1(R) -> Product8/1
  Add7/1 -> Reciprocal Sqrt4/1
  Asin2/1 -> [beta_back]
  Divide4/1 -> [miu_back]
  Gain3/1 -> Vector Concatenate8/1
  Reciprocal Sqrt5/1 -> MinMax2/1
  MinMax2/1 -> Divide5/2
  [i_n] -> H_to_Body_inv/1(i_n)
  Product1/1 -> Add/1
  Demux1/2 -> Product19/2, Product19/1
  Divide/1 -> [miu]
  [w_l] -> Product15/1
  Asin/1 -> [beta_rr]
  Bus Selector2/1 -> Vector Concatenate7/1  "<vx>"
  [w_r] -> Tw_r/1(In1)
  MinMax/1 -> Divide1/2
  Bus Selector1/6 -> Vector Concatenate5/1  "<wx>"
  Product10/1 -> Add3/2
  Add/1 -> Demux/1
  Constant20/1 -> locate_matrix3/1(xlr)
  Subsystem1/1(Hh_r) -> Gain/1
  Reciprocal Sqrt3/1 -> MinMax1/1
  Bus Selector3/8 -> Vector Concatenate/3  "<wz>"
  Tw_back/1(Tw_back) -> [Tb], Vector Concatenate8/2
  Vector Concatenate3/1 -> Product6/2
  Add5/1 -> Reciprocal Sqrt3/1
  Vector Concatenate6/1 -> Product11/2
  [w_r] -> Product5/1
  [state] -> Bus Selector2/1
  Demux1/3 -> Product20/1, Divide5/1, Product20/2
  Subsystem2/2(Sh_l) -> Gain2/1
  Vector Concatenate1/1 -> Product16/3
  Product13/1 -> Add4/2
  Bus Selector3/1 -> Vector Concatenate2/1  "<vx>"
  Reciprocal Sqrt/1 -> Divide/1
  Bus Selector1/7 -> Vector Concatenate5/2  "<wy>"
  Bus Selector3/6 -> Vector Concatenate/1  "<wx>"
  Bus Selector3/4 -> Scope1/1  "<gamma>"
  Vector Concatenate8/1 -> Product23/2, Fxyz_back/1
  Reciprocal Sqrt2/1 -> Divide2/1
  Divide1/1 -> Asin/1
  Bus Selector3/7 -> Vector Concatenate/2  "<wy>"
  Vector Concatenate4/1 -> Product8/2
  MinMax1/1 -> Divide3/2
  Demux2/3 -> Product14/1, Divide3/1, Product14/2
  locate_matrix7/1(R) -> Product9/1
  Add6/1 -> Demux1/1
  w_l/1 -> [w_r]
  Bus Selector3/3 -> Vector Concatenate2/3  "<vz>"
  [w_l] -> Sw_l/1(In1)
  Gain2/1 -> Vector Concatenate4/3
  Subsystem2/1(Hh_l) -> Gain1/1
  w_back/1 -> [w_back]
  Reciprocal Sqrt4/1 -> Divide4/1
  Constant12/1 -> MinMax/2
  Constant19/1 -> MinMax1/2
  Constant21/1 -> locate_matrix3/2(ylr)
  Bus Selector2/2 -> Vector Concatenate7/2  "<vy>"
  Product4/1 -> Add2/2, Add1/3
  Bus Selector3/2 -> Vector Concatenate2/2  "<vy>"
  locate_matrix/1(R) -> Product/2
  Product6/1 -> Product7/2, Fxyz_r/1
  Constant4/1 -> locate_matrix/1(xrr)
  Bus Selector2/4 -> Scope5/1  "<gamma>"
  Bus Selector2/6 -> Vector Concatenate1/1  "<wx>"
  Subsystem3/2(Sh_back) -> Vector Concatenate8/3
  Add3/1 -> Demux2/1
  Bus Selector1/8 -> Vector Concatenate5/3  "<wz>"
  Bus Selector2/7 -> Vector Concatenate1/2  "<wy>"
  [i_n] -> H_to_Body_inv1/1(i_n)
  Product9/1 -> Mxyz_l/1
  Vector Concatenate/1 -> Product/3
  Bus Selector1/5 -> Scope4/1  "<theta>"
  Product20/1 -> Add8/2, Add7/3
  i_n/1 -> [i_n]
  H_to_Body1/1(R) -> Product6/1
  Vector Concatenate7/1 -> Product17/2
  Product15/1 -> Divide2/2
  Asin1/1 -> [beta_lr]
  locate_matrix4/1(R) -> Product16/2
  Reciprocal Sqrt1/1 -> MinMax/1
  Constant6/1 -> locate_matrix/3(zrr)
  [w_l] -> Hw_l/1(In1)
  Constant27/1 -> locate_matrix4/3(z_back)
  Bus Selector1/1 -> Vector Concatenate6/1  "<vx>"
  Bus Selector1/2 -> Vector Concatenate6/2  "<vy>"
  Demux/1 -> Product2/2, Product2/1
  Vector Concatenate5/1 -> Product10/3
  [i_n] -> H_to_Body3/1(i_n)
  locate_matrix5/1(R) -> Product23/1
  Product23/1 -> Mxyz_back/1
  w_r/1 -> [w_l]
  [w_back] -> Product21/1
  Constant22/1 -> locate_matrix3/3(zlr)
  Bus Selector2/5 -> Scope6/1  "<theta>"
  Subsystem1/2(Sh_r) -> Vector Concatenate3/3
  [w_back] -> Sw_back/1(In1)
  Product5/1 -> Divide/2
  [i_n] -> H_to_Body_inv2/1(i_n)
  Constant25/1 -> locate_matrix4/1(x_back)
  Product17/1 -> Add6/1
  [i_n] -> H_to_Body1/1(i_n)
  H_to_Body_inv1/1(R) -> Product11/1, Product10/1
  Bus Selector1/4 -> Scope3/1  "<gamma>"
  Bus Selector3/5 -> Scope2/1  "<theta>"
  Demux2/2 -> Product13/2, Product13/1
  Gain1/1 -> Vector Concatenate4/1
  locate_matrix1/1(R) -> Product7/1
  Gain/1 -> Vector Concatenate3/1
  Constant8/1 -> MinMax2/2
  Product11/1 -> Add3/1
  Add1/1 -> Reciprocal Sqrt/1
  Product19/1 -> Add7/2
  Vector Concatenate2/1 -> Product1/2
  Product7/1 -> Mxyz_r/1
  [w_back] -> Tw_back/1(In1)
  H_to_Body_inv2/1(R) -> Product17/1, Product16/1
  Constant18/1 -> Product15/2
  [w_l] -> Tw_l/1(In1)
  Tw_r/1(Tw_r) -> [Tr], Vector Concatenate3/2
  Sw_back/1(Sw_back) -> Gain6/1
  Hw_back/1(Hw_back) -> Gain5/1
  Hw_r/1(Hw_r) -> Gain7/1
  Sw_r/1(Sw_r) -> Gain8/1
  Hw_l/1(Hw_l) -> Gain9/1
  Sw_l/1(Sw_l) -> Gain10/1
  Gain5/1 -> Subsystem3/1(Hw_back)
  Gain6/1 -> Subsystem3/2(Sw_back)
  Gain9/1 -> Subsystem2/1(Hw_l)
  Gain10/1 -> Subsystem2/2(Sw_l)
  Gain7/1 -> Subsystem1/1(Hw_r)
  Gain8/1 -> Subsystem1/2(Sw_r)
  Cos/1 -> Product22/1
  Constant14/1 -> Product22/2, Product24/2
  Product22/1 -> Sum/1
  Constant13/1 -> Sum/2
  Cos1/1 -> Product24/1
  Constant15/1 -> locate_matrix1/3(zrr)
  Product24/1 -> locate_matrix1/2(yrr)
  Sum/1 -> locate_matrix1/1(xrr)
  Cos2/1 -> Product25/1
  Cos3/1 -> Product29/1
  Constant16/1 -> Product25/2, Product29/2
  Constant3/1 -> Sum1/2
  Product25/1 -> Sum1/1
  [i_n] -> Cos1/1, Cos/1
  [i_n] -> Cos3/1, Cos2/1
  Constant17/1 -> locate_matrix7/3(zlr)
  Product29/1 -> locate_matrix7/2(ylr)
  Sum1/1 -> locate_matrix7/1(xlr)
  Constant23/1 -> locate_matrix5/2(y_back), Sum3/1
  Constant9/1 -> Sum2/1, locate_matrix5/1(x_back)
  [y_back] -> Sum3/2
  Sum4/1 -> Scope/3
  Constant24/1 -> locate_matrix5/3(z_back), Sum4/1
  [z_back] -> Sum4/2
  Sum2/1 -> Scope/1
  Sum3/1 -> Scope/2
  [x_back] -> Sum2/2

== system Triple_rotor_Tilerotor_model/Subsystem ==
  F : Inport
  M : Inport  Port=2
  i_n : Inport  Port=3
  Bus Creator1 : BusCreator  Inputs=9
  Bus Creator2 : BusCreator  Inputs=2
  Demux2 : Demux  Outputs=3
  Demux5 : Demux  Outputs=3
  Demux6 : Demux  Outputs=3
  Demux7 : Demux  Outputs=2
  Eular_angle_calculation : Subsystem
  Integrator{,1,3..6} (6 alike) : Integrator
  Integrator2 : Integrator  InitialConditionSource=external  InitialCondition=initial_vx
  Integrator7 : Integrator  InitialConditionSource=external  InitialCondition=initial_pitch
  Integrator8 : Integrator  InitialConditionSource=external
  Integrator9 : Integrator  InitialConditionSource=external  InitialCondition=initial_height
  Matrix Multiply : Product  Multiplication=Matrix(*)
  Terminator : Terminator
  angle_velocity_calculation : Subsystem
  rot2(pitch) : MATLABFcn  MATLABFcn=rot2(u)  OutputDimensions=[2 2]  Output1D=off
  velocity_calculation : Subsystem
  Out1 : Outport
  Out2 : Outport  Port=2
  tag scope: height=global
  wires:
  Matrix Multiply/1 -> Demux7/1
  Integrator4/1 -> Bus Creator1/9  "wz"
  M/1 -> angle_velocity_calculation/1(M)
  Integrator3/1 -> Bus Creator1/8  "wy"
  Demux6/1 -> Integrator8/1
  Integrator1/1 -> Bus Creator1/3  "vz"
  Integrator6/1 -> Bus Creator1/5  "psi"
  angle_velocity_calculation/1(Out1) -> Demux5/1
  Eular_angle_calculation/1(dEular_angle) -> Demux6/1
  Demux5/2 -> Integrator3/1
  Integrator2/1 -> Bus Creator2/1, Bus Creator1/1  "vx"
  Demux2/2 -> Integrator/1
  Integrator8/1 -> Bus Creator1/4  "gamma"
  Demux7/1 -> Terminator/1
  Demux2/3 -> Integrator1/1
  Demux2/1 -> Integrator2/1
  i_n/1 -> angle_velocity_calculation/2(i_n)
  Integrator7/1 -> rot2(pitch)/1, Bus Creator1/6  "theta"
  F/1 -> velocity_calculation/1(F)
  Bus Creator1/1 -> Out1/1
  Integrator/1 -> Bus Creator1/2, Bus Creator2/2  "vy"
  Demux6/3 -> Integrator7/1
  Demux5/1 -> Integrator5/1
  Integrator5/1 -> Bus Creator1/7  "wx"
  velocity_calculation/1(dv) -> Demux2/1
  rot2(pitch)/1 -> Matrix Multiply/1
  [initial_Vx] -> Integrator2/2
  Demux5/3 -> Integrator4/1
  Demux6/2 -> Integrator6/1
  Bus Creator2/1 -> Matrix Multiply/2
  Demux7/2 -> Integrator9/1
  [initial_height] -> Integrator9/2
  [initial_gamma] -> Integrator8/2
  [initial_theta] -> Integrator7/2
  Integrator9/1 -> Out2/1, [height]  "height"

== system Triple_rotor_Tilerotor_model/Vertical_Take_off ==
  Bus Creator : BusCreator  Inputs=4
  Constant : Constant  Value=Aerodynamic_switch
  Constant1 : Constant  Value=0
  Constant2 : Constant  Value=0
  Constant3 : Constant  Value=0
  Constant4 : Constant  Value=1e-5
  Ramp : simulink/Sources/Ramp  slope=slope_y  start=0  InitialOutput=0
  Saturation2 : Saturate  UpperLimit=max_y  LowerLimit=0
  dx* : Constant  Value=0
  gamma* : Constant  Value=0
  theta* : Constant  Value=0
  tag scope: Aerodynamic_switch=global, command=global, initial_Vx=global, initial_gamma=global, initial_height=global, initial_theta=global
  wires:
  theta*/1 -> Bus Creator/4  "theta*"
  Saturation2/1 -> Bus Creator/2  "height*"
  gamma*/1 -> Bus Creator/3  "gamma*"
  Ramp/1 -> Saturation2/1
  dx*/1 -> Bus Creator/1  "Vx*"
  Bus Creator/1 -> [command]
  Constant/1 -> [Aerodynamic_switch]
  Constant1/1 -> [initial_theta]
  Constant3/1 -> [initial_gamma]
  Constant2/1 -> [initial_height]
  Constant4/1 -> [initial_Vx]

== system Triple_rotor_Tilerotor_model/Vertical_descend ==
  Bus Creator : BusCreator  Inputs=4
  Constant : Constant  Value=Aerodynamic_switch
  Constant1 : Constant  Value=0
  Constant2 : Constant  Value=initial_y
  Constant3 : Constant  Value=0
  Constant4 : Constant  Value=1e-5
  Ramp : simulink/Sources/Ramp  slope=-slope_y  start=0  InitialOutput=initial_y
  Saturation2 : Saturate  UpperLimit=inf  LowerLimit=0
  dx* : Constant  Value=0
  gamma* : Constant  Value=0
  theta* : Constant  Value=0
  tag scope: Aerodynamic_switch=global, command=global, initial_Vx=global, initial_gamma=global, initial_height=global, initial_theta=global
  wires:
  theta*/1 -> Bus Creator/4  "theta*"
  Saturation2/1 -> Bus Creator/2  "height*"
  gamma*/1 -> Bus Creator/3  "gamma*"
  Ramp/1 -> Saturation2/1
  dx*/1 -> Bus Creator/1  "Vx*"
  Bus Creator/1 -> [command]
  Constant/1 -> [Aerodynamic_switch]
  Constant1/1 -> [initial_theta]
  Constant3/1 -> [initial_gamma]
  Constant2/1 -> [initial_height]
  Constant4/1 -> [initial_Vx]

== system Triple_rotor_Tilerotor_model/Vx ==
  Bus Creator : BusCreator  Inputs=4
  Constant : Constant  Value=Aerodynamic_switch
  Constant2 : Constant  Value=1000
  Constant4 : Constant  Value=100
  Constant5 : Constant  Value=4
  Constant6 : Constant  Value=0
  Gain : Gain  Gain=pi/180
  Gain1 : Gain  Gain=pi/180
  Ramp : simulink/Sources/Ramp  slope=slope  start=0  InitialOutput=100
  Saturation2 : Saturate  UpperLimit=final_velocity  LowerLimit=0
  gamma* : Constant  Value=0
  height : Constant  Value=1000
  theta* : Constant  Value=4
  tag scope: Aerodynamic_switch=global, command=global, initial_Vx=global, initial_gamma=global, initial_height=global, initial_theta=global
  wires:
  theta*/1 -> Bus Creator/4  "theta*"
  height/1 -> Bus Creator/2  "height*"
  gamma*/1 -> Bus Creator/3  "gamma*"
  Saturation2/1 -> Bus Creator/1  "Vx*"
  Bus Creator/1 -> [command]
  Constant/1 -> [Aerodynamic_switch]
  Constant2/1 -> [initial_height]
  Constant4/1 -> [initial_Vx]
  Ramp/1 -> Saturation2/1
  Gain/1 -> [initial_gamma]
  Constant6/1 -> Gain/1
  Gain1/1 -> [initial_theta]
  Constant5/1 -> Gain1/1

== system Triple_rotor_Tilerotor_model/angle_attack_control ==
  Bus Creator : BusCreator  Inputs=4
  Constant : Constant  Value=Aerodynamic_switch
  Constant2 : Constant  Value=1000
  Constant4 : Constant  Value=100
  Constant5 : Constant  Value=4
  Constant6 : Constant  Value=0
  Gain : Gain  Gain=pi/180
  Gain1 : Gain  Gain=pi/180
  Ramp : simulink/Sources/Ramp  slope=slope  start=0  InitialOutput=4
  Saturation2 : Saturate  UpperLimit=10  LowerLimit=final_theta
  dx* : Constant  Value=100
  gamma* : Constant  Value=0
  height : Constant  Value=1000
  tag scope: Aerodynamic_switch=global, command=global, initial_Vx=global, initial_gamma=global, initial_height=global, initial_theta=global
  wires:
  Saturation2/1 -> Bus Creator/4  "theta*"
  height/1 -> Bus Creator/2  "height*"
  gamma*/1 -> Bus Creator/3  "gamma*"
  dx*/1 -> Bus Creator/1  "Vx*"
  Bus Creator/1 -> [command]
  Constant/1 -> [Aerodynamic_switch]
  Constant2/1 -> [initial_height]
  Constant4/1 -> [initial_Vx]
  Gain/1 -> [initial_gamma]
  Constant6/1 -> Gain/1
  Gain1/1 -> [initial_theta]
  Constant5/1 -> Gain1/1
  Ramp/1 -> Saturation2/1
